simulink model "staticFreeplay"  (R2020b)
settings: Solver=VariableStepAuto  StartTime=0.0  StopTime=10.0  RelTol=1e-3
undefined symbols (not defined in the file): freeplay, stiffness
settings Model: Creator=Nicola Fonzi  LastModifiedBy=Nicola Fonzi

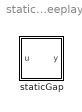
== system staticFreeplay ==
  staticGap : Subsystem

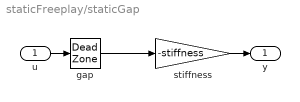
== system staticFreeplay/staticGap ==
  u : Inport
  gap : DeadZone  LowerValue=-freeplay  UpperValue=freeplay  SaturateOnIntegerOverflow=on
  stiffness : Gain  Gain=-stiffness
  y : Outport
  wires:
  u/1 -> gap/1
  stiffness/1 -> y/1
  gap/1 -> stiffness/1
